simulink model "Q5_observer"  (R2021b)
settings: Solver=VariableStepAuto  StartTime=0.0  StopTime=10.0  RelTol=1e-3
settings Model: Creator=user  LastModifiedBy=user

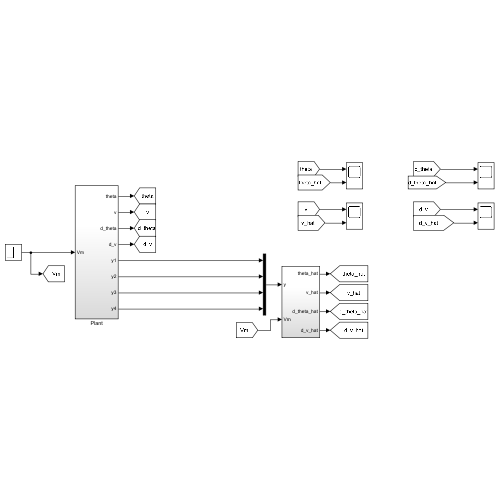
[thumbnail: Simulink's stored preview of the top-level diagram]
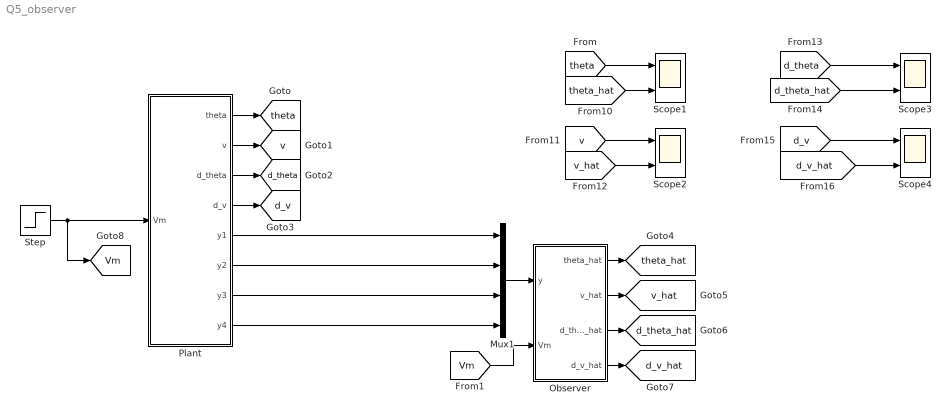
== system Q5_observer ==
  Mux1 : Mux
  Observer : Subsystem
  Plant : Subsystem
  Scope{1..4} (4 alike) : Scope  NumInputPorts=2
  Step : Step  Time=4  Before=2  After=8  SampleTime=0
  tag scope: Vm=global, d_theta=global, d_theta_hat=global, d_v=global, d_v_hat=global, theta=global, theta_hat=global, v=global, v_hat=global
  wires:
  [d_theta] -> Scope3/1
  [d_theta_hat] -> Scope3/2
  [Vm] -> Observer/2(Vm)
  Plant/1(theta) -> [theta]
  Observer/4(d_v_hat) -> [d_v_hat]
  [d_v] -> Scope4/1
  Mux1/1 -> Observer/1(y)
  Observer/3(d_theta_hat) -> [d_theta_hat]
  [theta_hat] -> Scope1/2
  [d_v_hat] -> Scope4/2
  [theta] -> Scope1/1
  Plant/8(y4) -> Mux1/4
  Plant/3(d_theta) -> [d_theta]
  Observer/1(theta_hat) -> [theta_hat]
  Plant/6(y2) -> Mux1/2
  Plant/2(v) -> [v]
  Plant/5(y1) -> Mux1/1
  [v_hat] -> Scope2/2
  [v] -> Scope2/1
  Observer/2(v_hat) -> [v_hat]
  Plant/4(d_v) -> [d_v]
  Step/1 -> [Vm], Plant/1(Vm)
  Plant/7(y3) -> Mux1/3

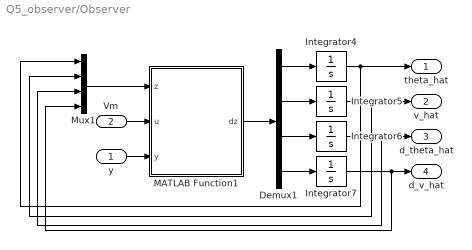
== system Q5_observer/Observer ==
  y : Inport
  Vm : Inport  Port=2
  Demux1 : Demux
  Integrator{4..7} (4 alike) : Integrator
  MATLAB Function1 : MATLAB Function  TreatAsAtomicUnit=on
  Mux1 : Mux
  theta_hat : Outport
  v_hat : Outport  Port=2
  d_theta_hat : Outport  Port=3
  d_v_hat : Outport  Port=4
  wires:
  MATLAB Function1/1(dz) -> Demux1/1
  Mux1/1 -> MATLAB Function1/1(z)
  Demux1/1 -> Integrator4/1
  Demux1/2 -> Integrator5/1
  Demux1/3 -> Integrator6/1
  Demux1/4 -> Integrator7/1
  Integrator5/1 -> Mux1/2, v_hat/1
  Integrator6/1 -> Mux1/3, d_theta_hat/1
  Integrator7/1 -> Mux1/4, d_v_hat/1
  y/1 -> MATLAB Function1/3(y)
  Integrator4/1 -> Mux1/1, theta_hat/1
  Vm/1 -> MATLAB Function1/2(u)

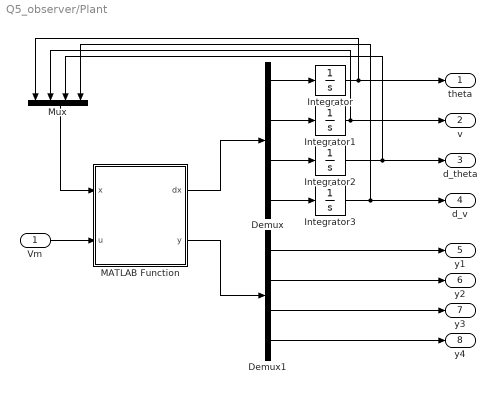
== system Q5_observer/Plant ==
  Vm : Inport
  Demux : Demux
  Demux1 : Demux
  Integrator{,1..3} (4 alike) : Integrator
  MATLAB Function : MATLAB Function  TreatAsAtomicUnit=on
  Mux : Mux
  theta : Outport
  v : Outport  Port=2
  d_theta : Outport  Port=3
  d_v : Outport  Port=4
  y1 : Outport  Port=5
  y2 : Outport  Port=6
  y3 : Outport  Port=7
  y4 : Outport  Port=8
  wires:
  Vm/1 -> MATLAB Function/2(u)
  Mux/1 -> MATLAB Function/1(x)
  Demux/1 -> Integrator/1
  Demux/2 -> Integrator1/1
  Demux/3 -> Integrator2/1
  Demux/4 -> Integrator3/1
  Integrator/1 -> theta/1, Mux/1
  Integrator1/1 -> v/1, Mux/2
  Integrator2/1 -> d_theta/1, Mux/3
  Integrator3/1 -> d_v/1, Mux/4
  MATLAB Function/1(dx) -> Demux/1
  Demux1/1 -> y1/1
  Demux1/2 -> y2/1
  Demux1/3 -> y3/1
  Demux1/4 -> y4/1
  MATLAB Function/2(y) -> Demux1/1

== matlab function Q5_observer/Observer/MATLAB Function1 ==
  data: z input; u input; y input; dz output
function dz = observer(z,u,y)
dz = zeros(4,1);
A = [0 0 1 0;0 0 0 1;0 483.1312 -28.2625 0;0 -837.2130 28.2625 0];
B = [0;0;49.7076;-49.7076];
C = eye(4);
L_p = [5 -1 1 0;1 5 0 1;0 483.1312 -20.2625 -0.5;0 -837.213 28.7625 8];
temp = (A-L_p*C)*z;
temp2 = B*u;
temp3 = L_p*y;
dz = temp(:,1)+temp2(:,1)+temp3(:,1);
end

== matlab function Q5_observer/Plant/MATLAB Function ==
  data: dx output; y output; x input; u input
function [dx, y] = plant(x,u)
dx = zeros(4,1);
A = [0 0 1 0;0 0 0 1;0 483.1312 -28.2625 0;0 -837.2130 28.2625 0];
B = [0;0;49.7076;-49.7076];
C = eye(4);
temp = A*x;
temp2 = B*u;
dx = temp(:,1) + temp2(:,1);
y = C*x;
%y = size(dx,1);
end
